simulink model "ExampleOpponentTelemetry"  (Simulink 9.2)
settings: Solver=FixedStepDiscrete  StartTime=0.0  StopTime=inf  FixedStep=0.001  RelTol=1e-3  EnableMultiTasking=on
PostLoadFcn:
  | TIMESTEP = 0.001;
libraries: rFproPhysicsLib x7, simulink x1
settings Model: Creator=enewton  LastModifiedBy=SeanKavanagh
settings Model: SuppressorTable=|
  | <?xml version="1.0" encoding="UTF-8" standalone="yes" ?>
  | <!DOCTYPE boost_serialization>
  | <boost_serialization signature="serialization::archive" version="15">
  | <DiagnosticSuppressor class_id="0" tracking_level="0" version="6">
  | 	<Table class_id="1" tracking_level="0" version="0">
  | 		<count>2</count>
  | 		<bucket_count>8</bucket_count>
  | 		<item_version>0</item_version>
  | 		<item class_id="2" tracking_level="0" version="0">
  | 			<first class_id="3" tracking_level="0" version="6">
  | 				<Source class_id="4" tracking_level="0" version="0">
  | 					<count>1</count>
  | 					<item_version>0</item_version>
  | 					<item>ExampleOpponentTelemetry/Additional Vehicle/Send Enable/Subsystem/Counter Free-Running2</item>
  | 				</Source>
  | 			</first>
  | 			<second class_id="5" tracking_level="0" version="6">
  | 				<SuppressedData class_id="6" tracking_level="0" version="0">
  | 					<count>2</count>
  | 					<bucket_count>8</bucket_count>
  | 					<item_version>0</item_version>
  | 					<item class_id="7" tracking_level="0" version="0">
  | 						<first class_id="8" tracking_level="0" version="6">
  | 							<ID>SimulinkFixedPoint:util:Overflowoccurred</ID>
  | 							<Cause>
  | 								<Source>
  | 									<count>0</count>
  | 									<item_version>0</item_version>
  | 								</Source>
  | 							</Cause>
  | 						</first>
  | 						<second class_id="9" tracking_level="0" version="6">
  | 							<Comment></Comment>
  | 							<User></User>
  | 							<LastModified class_id="10" tracking_level="0" version="0">
  | 								<ptime_date class_id="11" tracking_level="0" version="0">
  | 									<date>20160523</date>
  | 								</ptime_date>
  | 								<ptime_time_duration class_id="12" tracking_level="0" version="0">
  | 									<is_special>0</is_special>
  | 									<time_duration_hours>10</time_duration_hours>
  | 									<time_duration_minutes>57</time_duration_minutes>
  | 									<time_duration_seconds>55</time_duration_seconds>
  | 									<time_duration_fractional_seconds>0</time_duration_fractional_seconds>
  | 								</ptime_time_duration>
  | 							</LastModified>
  | 							<SuppressionType>1</SuppressionType>
  | 						</second>
  | 					</item>
  | 					<item>
  | 						<first>
  | 							<ID>Simulink:DataType:WarningOverFlowDetected</ID>
  | 							<Cause>
  | 								<Source>
  | 									<count>0</count>
  | 									<item_version>0</item_version>
  | 								</Source>
  | 							</Cause>
  | 						</first>
  | 						<second>
  | 							<Comment></Comment>
  | 							<User></User>
  | 							<LastModified>
  | 								<ptime_date>
  | 									<date>20160523</date>
  | 								</ptime_date>
  | 								<ptime_time_duration>
  | 									<is_special>0</is_special>
  | 									<time_duration_hours>10</time_duration_hours>
  | 									<time_duration_minutes>57</time_duration_minutes>
  | 									<time_duration_seconds>55</time_duration_seconds>
  | 									<time_duration_fractional_seconds>0</time_duration_fractional_seconds>
  | 								</ptime_time_duration>
  | 							</LastModified>
  | 							<SuppressionType>1</SuppressionType>
  | 						</second>
  | 					</item>
  | 				</SuppressedData>
  | 			</second>
  | 		</item>
  | 		<item>
  | 			<first>
  | 				<Source>
  | 					<count>1</count>
  | 					<item_version>0</item_version>
  | 					<item>ExampleOpponentTelemetry/Additional Vehicle1/Send Enable/Subsystem/Counter Free-Running2</item>
  | 				</Source>
  | 			</first>
  | 			<second>
  | 				<SuppressedData>
  | 					<count>2</count>
  | 					<bucket_count>8</bucket_count>
  | 					<item_version>0</item_version>
  | 					<item>
  | 						<first>
  | 							<ID>SimulinkFixedPoint:util:Overflowoccurred</ID>
  | 							<Cause>
  | 								<Source>
  | 									<count>0</count>
  | 									<item_version>0</item_version>
  | 								</Source>
  | 							</Cause>
  | 						</first>
  | 						<second>
  | 							<Comment></Comment>
  | 							<User></User>
  | 							<LastModified>
  | 								<ptime_date>
  | 									<date>20160523</date>
  | 								</ptime_date>
  | 								<ptime_time_duration>
  | 									<is_special>0</is_special>
  | 									<time_duration_hours>10</time_duration_hours>
  | 									<time_duration_minutes>57</time_duration_minutes>
  | 									<time_duration_seconds>55</time_duration_seconds>
  | 									<time_duration_fractional_seconds>0</time_duration_fractional_seconds>
  | 								</ptime_time_duration>
  | 							</LastModified>
  | 							<SuppressionType>1</SuppressionType>
  | 						</second>
  | 					</item>
  | 					<item>
  | 						<first>
  | 							<ID>Simulink:DataType:WarningOverFlowDetected</ID>
  | 							<Cause>
  | 								<Source>
  | 									<count>0</count>
  | 									<item_version>0</item_version>
  | 								</Source>
  | 							</Cause>
  | 						</first>
  | 						<second>
  | 							<Comment></Comment>
  | 							<User></User>
  | 							<LastModified>
  | 								<ptime_date>
  | 									<date>20160523</date>
  | 								</ptime_date>
  | 								<ptime_time_duration>
  | 									<is_special>0</is_special>
  | 									<time_duration_hours>10</time_duration_hours>
  | 									<time_duration_minutes>57</time_duration_minutes>
  | 									<time_duration_seconds>55</time_duration_seconds>
  | 									<time_duration_fractional_seconds>0</time_duration_fractional_seconds>
  | 								</ptime_time_duration>
  | 							</LastModified>
  | 							<SuppressionType>1</SuppressionType>
  | 						</second>
  | 					</item>
  | 				</SuppressedData>
  | 			</second>
  | 		</item>
  | 	</Table>
  | </DiagnosticSuppressor>
  | </boost_serialization>
settings OptimizationCC: ExpressionDepthLimit=2147483647
settings DebuggingCC: SolverPrmCheckMsg=warning
settings RTWCC: SystemTargetFile=rfpro.tlc  MakeCommand="make_rtw OPTS=\"-DRUN_PHYSICS\""  TemplateMakefile=rfpro.tmf  Description=rFpro Target (Run Physics)  TargetLang=C++
settings STFCustomTargetCC: ModelReferenceCompliant=off  GeneratePreprocessorConditionals=Disable all  CombineOutputUpdateFcns=on  MatFileLogging=on  CPPClassGenCompliant=on  GRTInterface=off  SystemTargetFile=rfpro.tlc
settings GRTTargetCC: ModelReferenceCompliant=off  ParMdlRefBuildCompliant=off  CompOptLevelCompliant=off  ConcurrentExecutionCompliant=off  CombineOutputUpdateFcns=on  GRTInterface=off  UseToolchainInfoCompliant=off

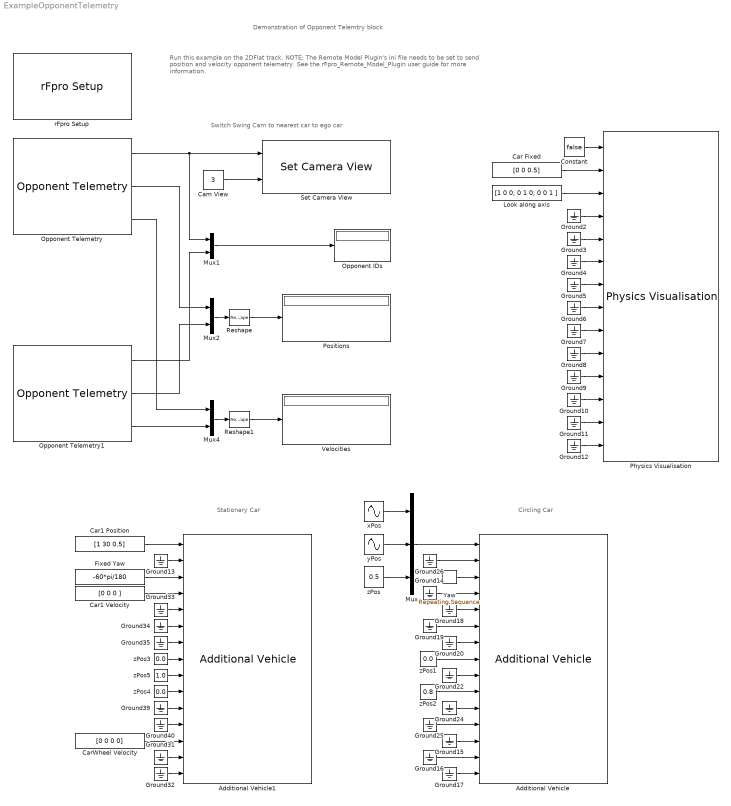
== system ExampleOpponentTelemetry ==
  note: Run this example on the 2DFlat track.
      |
      | NOTE: The Remote Model Plugin's ini file needs to be set to send position and velocity opponent telemetry.
      | See the rFpro_Remote_Model_Plugin user guide for more information.
  note: Switch Swing Cam to nearest car to ego car
  note: Circling Car
  note: Stationary Car
  note: Demonstration of Opponent Telemtry block
  Additional Vehicle : rFproPhysicsLib/Additional Vehicle  VEH_FILE='Hatchback_AWD_Blue'  DRIVER_NAME=''  UPGRADE_PACK=0  SKIN=''  HELMET=''  COLLIDABLE=off  TRANSPARENT_PROXIMITY=0  MANUAL_TRANSPARENCY=0  HEIGHT_VALID=on  ORI_VALID=off  HEADING_VALID=on  VEL_VALID=off  ROT_VALID=off  GEAR_VALID=off  RPM_VALID=off  INPUTS_VALID=on  BRAKE_LIGHT_VALID=off  HEADLIGHT_VALID=off  WHEEL_ROTATIONS_VALID=off  WHEEL_BRAKE_TEMPS_VALID=off  WHEEL_HEIGHTS_VALID=off  period=0.01  offset=0  useReverseByteOrder=on  rFpro__platform=Remote Model - Default
  Additional Vehicle1 : rFproPhysicsLib/Additional Vehicle  VEH_FILE='Hatchback_AWD_White'  DRIVER_NAME=''  UPGRADE_PACK=0  SKIN=''  HELMET=''  COLLIDABLE=off  TRANSPARENT_PROXIMITY=0  MANUAL_TRANSPARENCY=0  HEIGHT_VALID=on  ORI_VALID=off  HEADING_VALID=on  VEL_VALID=on  ROT_VALID=off  GEAR_VALID=off  RPM_VALID=off  INPUTS_VALID=on  BRAKE_LIGHT_VALID=off  HEADLIGHT_VALID=off  WHEEL_ROTATIONS_VALID=on  WHEEL_BRAKE_TEMPS_VALID=off  WHEEL_HEIGHTS_VALID=off  period=0.01  offset=0  useReverseByteOrder=on  rFpro__platform=Remote Model - Default
  Cam View : Constant  Value=3
  Car Fixed : Constant  Value=[0 0 0.5]
  Car1 Position : Constant  Value=[1 30 0.5]
  Car1 Velocity : Constant  Value=[0 0 0 ]
  CarWheel Velocity : Constant  Value=[0 0 0 0]
  Constant : Constant  Value=false
  Fixed Yaw : Constant  Value=-60*pi/180
  Ground{2..20,22,24..26,31..35,39..40} (30 alike) : Ground
  Look along axis : Constant  Value=[1 0 0; 0 1 0; 0 0 1 ]
  Mux : Mux  Inputs=3
  Mux1 : Mux  Inputs=2
  Mux2 : Mux  Inputs=2
  Mux4 : Mux  Inputs=2
  Opponent IDs : Display
  Opponent Telemetry : rFproPhysicsLib/Opponent Telemetry  veh_select=Nth Nearest  veh_id=0  ext_id=off  rFpro__platform=Remote Model - Default  pick_Veh_ID=on  pick_Lap=off  pick_Gear=off  pick_Sector=off  pick_Vis_Wheel_Range=off  pick_PG_Offset=off  pick_Phys_Wheel_Range=off  pick_Standard_Location=off  pick_Brake_Torque=off  pick_sLap_Ref=off  pick_DT=off  pick_ET=off  pick_LapStart=off  pick_Pos=on  pick_Vel=on  pick_Accel=off  pick_Ori=off  pick_Rot=off  pick_RotAccel=off  pick_RPM=off  pick_WaterT=off  pick_OilT=off  pick_Clutch_RPM=off  pick_UF_Throttle=off  pick_UF_Brake=off  pick_UF_Steer=off  pick_UF_Clutch=off  pick_F_Throttle=off  pick_F_Brake=off  pick_F_Steer=off  pick_F_Clutch=off  pick_Steer_F=off  pick_F3_Move=off  pick_R3_Move=off  pick_F_Wing=off  pick_F_Ride=off  pick_R_Ride=off  pick_Drag=off  pick_F_Down_F=off  pick_R_Down_F=off  pick_Fuel=off  pick_Max_RPM=off  pick_Impact_ET=off  pick_Impact_Mag=off  pick_Impact_Pos=off  pick_Engine_Torque=off  pick_Fuel_capacity=off  pick_R_Brake_Bias=off  pick_Turbo_P=off  pick_Lap_Dist=off  pick_Dist_To_Groove=off  pick_Stops=off  pick_Overheating=off  pick_Detached=off  pick_Headlights=off  pick_Dent_Severity=off  pick_Speed_Limiter=off  pick_Max_Gears=off  pick_FT_Compound_idx=off  pick_RT_Compound_idx=off  pick_F_Flap=off  pick_R_Flap=off  pick_Ig_Starter=off  pick_Have_Speed_Limiter=off  pick_Anti_Stall_Active=off  pick_Beacons=off
  Opponent Telemetry1 : rFproPhysicsLib/Opponent Telemetry  veh_select=Nth Nearest  veh_id=1  ext_id=off  rFpro__platform=Remote Model - Default  pick_Veh_ID=on  pick_Lap=off  pick_Gear=off  pick_Sector=off  pick_Vis_Wheel_Range=off  pick_PG_Offset=off  pick_Phys_Wheel_Range=off  pick_Standard_Location=off  pick_Brake_Torque=off  pick_sLap_Ref=off  pick_DT=off  pick_ET=off  pick_LapStart=off  pick_Pos=on  pick_Vel=on  pick_Accel=off  pick_Ori=off  pick_Rot=off  pick_RotAccel=off  pick_RPM=off  pick_WaterT=off  pick_OilT=off  pick_Clutch_RPM=off  pick_UF_Throttle=off  pick_UF_Brake=off  pick_UF_Steer=off  pick_UF_Clutch=off  pick_F_Throttle=off  pick_F_Brake=off  pick_F_Steer=off  pick_F_Clutch=off  pick_Steer_F=off  pick_F3_Move=off  pick_R3_Move=off  pick_F_Wing=off  pick_F_Ride=off  pick_R_Ride=off  pick_Drag=off  pick_F_Down_F=off  pick_R_Down_F=off  pick_Fuel=off  pick_Max_RPM=off  pick_Impact_ET=off  pick_Impact_Mag=off  pick_Impact_Pos=off  pick_Engine_Torque=off  pick_Fuel_capacity=off  pick_R_Brake_Bias=off  pick_Turbo_P=off  pick_Lap_Dist=off  pick_Dist_To_Groove=off  pick_Stops=off  pick_Overheating=off  pick_Detached=off  pick_Headlights=off  pick_Dent_Severity=off  pick_Speed_Limiter=off  pick_Max_Gears=off  pick_FT_Compound_idx=off  pick_RT_Compound_idx=off  pick_F_Flap=off  pick_R_Flap=off  pick_Ig_Starter=off  pick_Have_Speed_Limiter=off  pick_Anti_Stall_Active=off  pick_Beacons=off
  Physics Visualisation : rFproPhysicsLib/Physics Visualisation  PAR_SKIP_INTERNAL_PHYSICS=off  PAR_ACCEL_VALID=off  PAR_ROT_ACCEL_VALID=off  PAR_GEAR_VALID=off  PAR_RPM_VALID=off  PAR_INPUTS_VALID=off  PAR_STEER_TORQUE_VALID=off  PAR_HEADLIGHTS_ON_VALID=off  PAR_WHEEL_POS_VALID=off  PAR_WHEEL_ORI_VALID=off  PAR_TYRE_PARAMS_VALID=off  PAR_WHEEL_ROTATION_VALID=off  PAR_WHEEL_BRAKE_TEMP_VALID=off  PAR_WHEEL_TREAD_TEMP_VALID=off  PAR_WHEEL_AIR_TEMP_VALID=off  period=-1  offset=0  useReverseByteOrder=on  rFpro__platform=Remote Model - Default
  Positions : Display
  Reshape : Reshape  OutputDimensionality=Customize  OutputDimensions=[3,2]
  Reshape1 : Reshape  OutputDimensionality=Customize  OutputDimensions=[3,2]
  Set Camera View : rFproPhysicsLib/Set Camera View  triggerWidth=1  useReverseByteOrder=off  rFpro__platform=Remote Model - Default
  Velocities : Display
  Yaw : simulink/Sources/Repeating Sequence  rep_seq_t=[0 6]  rep_seq_y=[0 -2*pi]
  rFpro Setup : rFproPhysicsLib/rFpro Setup  platform=Remote Model - Default  stopOnSessionEnd=on  usePseudoRealtime=on  syncToRF=on  useReverseByteOrder=off  useRfTime=on  minIterations=4  maxIterations=1000  ipReceiveAddress='127.0.0.1'  ipReceivePort=11054  receiveSampleTime=-1  ipTransmitAddress='127.0.0.1'  ipTransmitPort=11052  transmitSampleTime=-1  pluginType=RUN_PHYSICS  sysTarget=xpctarget.tlc  templateMakeFile=xpc_default_tmf  makeCommand=make_rtw  buildDesc=xPC target
  xPos : Sin  Amplitude=20  Bias=30  Frequency=2*pi/6  SampleTime=0
  yPos : Sin  Amplitude=20  Frequency=2*pi/6  Phase=pi/2  SampleTime=0
  zPos : Constant  Value=0.5
  zPos1 : Constant  Value=0.0
  zPos2 : Constant  Value=0.8
  zPos3 : Constant  Value=0.0
  zPos4 : Constant  Value=0.0
  zPos5 : Constant  Value=1.0
  wires:
  Constant/1 -> Physics Visualisation/1
  Car Fixed/1 -> Physics Visualisation/2
  Look along axis/1 -> Physics Visualisation/3
  Ground2/1 -> Physics Visualisation/4
  Ground3/1 -> Physics Visualisation/5
  Ground4/1 -> Physics Visualisation/6
  Ground5/1 -> Physics Visualisation/7
  Ground6/1 -> Physics Visualisation/8
  Ground7/1 -> Physics Visualisation/9
  Ground8/1 -> Physics Visualisation/10
  Ground9/1 -> Physics Visualisation/11
  Ground10/1 -> Physics Visualisation/12
  Ground11/1 -> Physics Visualisation/13
  Ground12/1 -> Physics Visualisation/14
  Ground17/1 -> Additional Vehicle/15
  Ground16/1 -> Additional Vehicle/14
  Ground15/1 -> Additional Vehicle/13
  Ground25/1 -> Additional Vehicle/12
  Ground24/1 -> Additional Vehicle/11
  zPos2/1 -> Additional Vehicle/10
  Ground22/1 -> Additional Vehicle/9
  zPos1/1 -> Additional Vehicle/8
  Ground20/1 -> Additional Vehicle/7
  Ground19/1 -> Additional Vehicle/6
  Ground18/1 -> Additional Vehicle/5
  Ground14/1 -> Additional Vehicle/4
  Yaw/1 -> Additional Vehicle/3
  Mux/1 -> Additional Vehicle/1
  Ground32/1 -> Additional Vehicle1/15
  Ground31/1 -> Additional Vehicle1/14
  CarWheel Velocity/1 -> Additional Vehicle1/13
  Ground40/1 -> Additional Vehicle1/12
  Ground39/1 -> Additional Vehicle1/11
  zPos4/1 -> Additional Vehicle1/10
  zPos5/1 -> Additional Vehicle1/9
  zPos3/1 -> Additional Vehicle1/8
  Ground35/1 -> Additional Vehicle1/7
  Ground34/1 -> Additional Vehicle1/6
  Ground33/1 -> Additional Vehicle1/5
  Car1 Velocity/1 -> Additional Vehicle1/4
  Fixed Yaw/1 -> Additional Vehicle1/3
  Car1 Position/1 -> Additional Vehicle1/1
  xPos/1 -> Mux/1
  yPos/1 -> Mux/2
  zPos/1 -> Mux/3
  Ground26/1 -> Additional Vehicle/2
  Cam View/1 -> Set Camera View/2
  Opponent Telemetry/1 -> Mux1/1, Set Camera View/1
  Ground13/1 -> Additional Vehicle1/2
  Opponent Telemetry1/1 -> Mux1/2
  Mux1/1 -> Opponent IDs/1
  Mux2/1 -> Reshape/1
  Opponent Telemetry/2 -> Mux2/1
  Opponent Telemetry1/2 -> Mux2/2
  Mux4/1 -> Reshape1/1
  Opponent Telemetry1/3 -> Mux4/2
  Opponent Telemetry/3 -> Mux4/1
  Reshape/1 -> Positions/1
  Reshape1/1 -> Velocities/1
